simulink model "num1new"  (R2018b)
settings: Solver=FixedStepAuto  StartTime=0.0  StopTime=10.0  FixedStep=0.025  RelTol=1e-3
values from neighbouring files (symbols this model uses):
  initialstate1 = 1    [num1a.m]    (also in num1b.m; num1c.m; num1d.m)
  initialstate2 = 0    [num1a.m]    (also in num1b.m; num1c.m; num1d.m = 1)
  initialstate3 = 0    [num1a.m]    (also in num1b.m; num1c.m; num1d.m = 1)
  tfinal = CL_final(end)    [num1a.m]    (also in num1b.m; num1c.m; num1d.m; num2a.m)
settings Model: Creator=reema  LastModifiedBy=reema

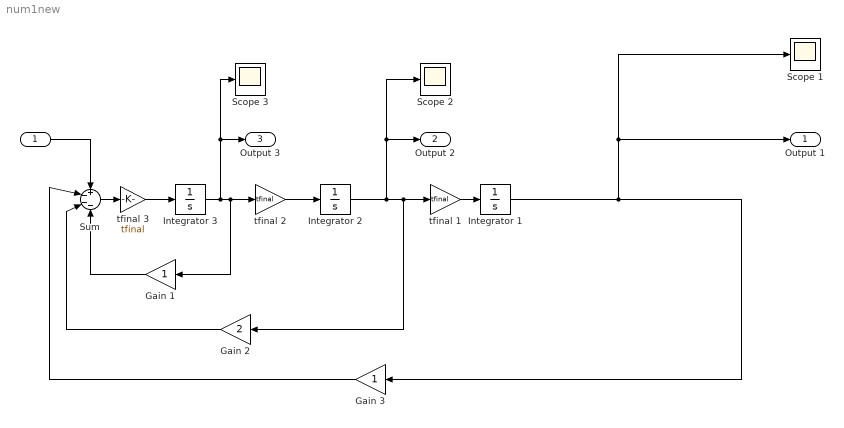
== system num1new ==
  " " : Inport
  " Integrator 3" : Integrator  InitialCondition=initialstate3
  Gain 1 : Gain
  Gain 2 : Gain  Gain=2
  Gain 3 : Gain
  Integrator 1 : Integrator  InitialCondition=initialstate1  UpperSaturationLimit=1  LowerSaturationLimit=-1
  Integrator 2 : Integrator  InitialCondition=initialstate2
  Scope 1 : Scope
  Scope 2 : Scope
  Scope 3 : Scope
  Sum : Sum  Inputs=+---
  "tfinal 1 " : Gain  Gain=tfinal
  tfinal 2 : Gain  Gain=tfinal
  tfinal 3 : Gain  Gain=tfinal
  Output 1 : Outport
  Output 2 : Outport  Port=2
  Output 3 : Outport  Port=3
  wires:
  "tfinal 1 "/1 -> Integrator 1/1
  Gain 1/1 -> Sum/4
  Integrator 2/1 -> "tfinal 1 "/1, Gain 2/1, Scope 2/1, Output 2/1
  Gain 2/1 -> Sum/3
  Sum/1 -> tfinal 3/1
  tfinal 3/1 -> " Integrator 3"/1
  tfinal 2/1 -> Integrator 2/1
  " "/1 -> Sum/1
  Gain 3/1 -> Sum/2
  Integrator 1/1 -> Output 1/1, Scope 1/1, Gain 3/1
  " Integrator 3"/1 -> Output 3/1, Scope 3/1, tfinal 2/1, Gain 1/1
